simulink model "test_SOC_SOH_multi_cell"  (R2024a)
settings: Solver=FixedStepAuto  StartTime=0.0  StopTime=3600*24*365  FixedStep=1  RelTol=1e-3
values from neighbouring files (symbols this model uses):
  SOH_ESTIM_INIT = 1.0    [SOXDictionaryGotion.sldd]
libraries: simulink x3
settings Model: DataDictionary=SOXDictionaryGotion.sldd  Creator=mmackenzie  LastModifiedBy=mmackenzie
settings OptimizationCC: DefaultUnderspecifiedDataType=single
settings DebuggingCC: ParamPrecisionLossAbsoluteDiffThreshold=1e-10  ParamPrecisionLossRelativeDiffThreshold=1e-6  AllowSymbolicDim=off

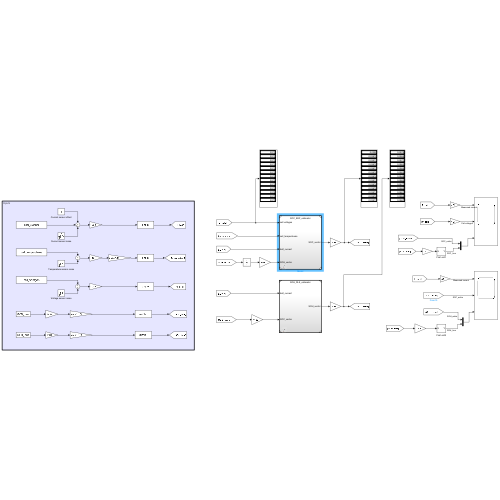
[thumbnail: Simulink's stored preview of the top-level diagram]
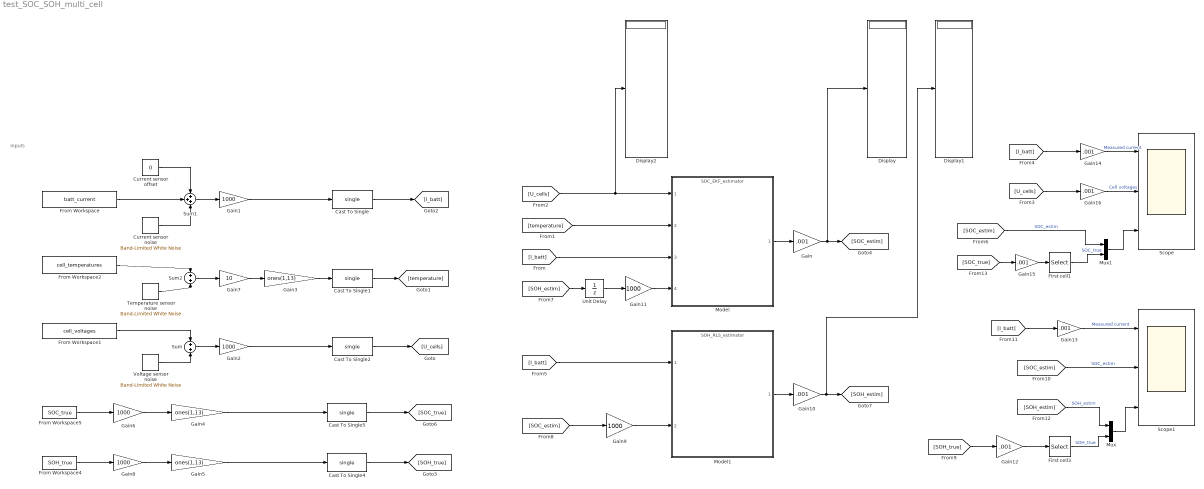
== system test_SOC_SOH_multi_cell ==
  note: Inputs
  Cast To Single{,1..2,4..5} (5 alike) : DataTypeConversion  OutDataTypeStr=single  SaturateOnIntegerOverflow=off  RndMeth=Floor
  Current sensor noise : simulink/Sources/Band-Limited White Noise  Cov=.1  Ts=1  seed=42
  Current sensor offset : Constant  Value=0
  Display : Display
  Display1 : Display
  Display2 : Display
  First cell1 : Selector  InputPortWidth=13  IndexOptions=Index vector (dialog)  Indices=1  OutputSizes=1
  First cell3 : Selector  InputPortWidth=13  IndexOptions=Index vector (dialog)  Indices=1  OutputSizes=1
  From Workspace : FromWorkspace  VariableName=batt_current
  From Workspace1 : FromWorkspace  VariableName=cell_voltages
  From Workspace2 : FromWorkspace  VariableName=cell_temperatures
  From Workspace4 : FromWorkspace  VariableName=SOH_true
  From Workspace5 : FromWorkspace  VariableName=SOC_true
  Gain{,10,12..16} (7 alike) : Gain  Gain=.001
  Gain{1..2,6,8..9,11} (6 alike) : Gain  Gain=1000
  Gain3 : Gain  Gain=ones(1,13)
  Gain4 : Gain  Gain=ones(1,13)
  Gain5 : Gain  Gain=ones(1,13)
  Gain7 : Gain  Gain=10
  Model : ModelReference  ModelNameDialog=SOC_EKF_estimator.slx  SimulationMode=Normal  ModelReferenceVersion=1.42
  Model1 : ModelReference  ModelNameDialog=SOH_RLS_estimator.slx  SimulationMode=Normal  ModelReferenceVersion=1.43
  Mux : Mux  Inputs=2
  Mux1 : Mux  Inputs=2
  Scope : Scope  NumInputPorts=3
  Scope1 : Scope  NumInputPorts=3
  Sum : Sum
  Sum1 : Sum  Inputs=+++
  Sum2 : Sum
  Temperature sensor noise : simulink/Sources/Band-Limited White Noise  Cov=1  Ts=1  seed=42
  Unit Delay : UnitDelay  InitialCondition=SOH_ESTIM_INIT  SampleTime=-1  HasFrameUpgradeWarning=on
  Voltage sensor noise : simulink/Sources/Band-Limited White Noise  Cov=1e-6  Ts=1  seed=42
  wires:
  [U_cells] -> Display2/1, Model/1
  [I_batt] -> Gain14/1
  Model/1 -> Gain/1
  From Workspace2/1 -> Sum2/1
  From Workspace/1 -> Sum1/2
  Sum2/1 -> Gain7/1
  Current sensor offset/1 -> Sum1/1
  From Workspace1/1 -> Sum/1
  Sum/1 -> Gain2/1
  Temperature sensor noise/1 -> Sum2/2
  Sum1/1 -> Gain1/1
  Current sensor noise/1 -> Sum1/3
  Voltage sensor noise/1 -> Sum/2
  [SOH_estim] -> Unit Delay/1
  [temperature] -> Model/2
  [I_batt] -> Model/3
  Gain/1 -> Display/1, [SOC_estim]
  Gain1/1 -> Cast To Single/1
  Gain7/1 -> Gain3/1
  Gain2/1 -> Cast To Single2/1
  Cast To Single/1 -> [I_batt]
  Cast To Single1/1 -> [temperature]
  Cast To Single2/1 -> [U_cells]
  [U_cells] -> Gain16/1
  Cast To Single4/1 -> [SOH_true]
  Gain5/1 -> Cast To Single4/1
  From Workspace5/1 -> Gain6/1
  Cast To Single5/1 -> [SOC_true]
  Gain8/1 -> Gain5/1
  From Workspace4/1 -> Gain8/1
  Gain6/1 -> Gain4/1
  Gain4/1 -> Cast To Single5/1
  [SOC_estim] -> Gain9/1
  Gain9/1 -> Model1/2
  [I_batt] -> Model1/1
  Gain10/1 -> Display1/1, [SOH_estim]
  Model1/1 -> Gain10/1
  Unit Delay/1 -> Gain11/1
  [SOC_estim] -> Scope1/2  "SOC_estim"
  Gain12/1 -> First cell3/1
  Mux/1 -> Scope1/3
  [SOH_true] -> Gain12/1
  [I_batt] -> Gain13/1
  Gain13/1 -> Scope1/1  "Measured current"
  Gain3/1 -> Cast To Single1/1
  [SOC_true] -> Gain15/1
  Mux1/1 -> Scope/3
  Gain15/1 -> First cell1/1
  Gain14/1 -> Scope/1  "Measured current"
  Gain16/1 -> Scope/2  "Cell voltages"
  [SOC_estim] -> Mux1/1  "SOC_estim"
  First cell1/1 -> Mux1/2  "SOC_true"
  [SOH_estim] -> Mux/1  "SOH_estim"
  First cell3/1 -> Mux/2  "SOH_true"
  Gain11/1 -> Model/4
